simulink model "PV_RT_PI_2017b"  (R2017b)
settings: Solver=ode23tb  StartTime=0.0  StopTime=30  FixedStep=0.01  RelTol=1e-3
values from neighbouring files (symbols this model uses):
  a1 = 900    [LFC_PV_Test_System_Parameters.m]
  B1 = 0.8    [LFC_PV_Test_System_Parameters.m]
  b1 = -18    [LFC_PV_Test_System_Parameters.m]
  c1 = 100    [LFC_PV_Test_System_Parameters.m]
  d1 = 50    [LFC_PV_Test_System_Parameters.m]
  Kps1 = 120    [LFC_PV_Test_System_Parameters.m]
  Kr1 = 0.33    [LFC_PV_Test_System_Parameters.m]
  R1 = 2.5    [LFC_PV_Test_System_Parameters.m]
  T12 = 0.545    [LFC_PV_Test_System_Parameters.m]
  Tg1 = 0.08    [LFC_PV_Test_System_Parameters.m]
  Tps1 = 20    [LFC_PV_Test_System_Parameters.m]
  Tr1 = 10    [LFC_PV_Test_System_Parameters.m]
  Tt1 = 0.3    [LFC_PV_Test_System_Parameters.m]
undefined symbols (not defined in the file or in its folder): Kd, Ki1, Ki2, Kp1, Kp2
libraries: simulink x2
settings Model: Creator=Fujitsu  LastModifiedBy=bora_
settings SolverCC: ZeroCrossAlgorithm=Adaptive
settings DataIOCC: MaxDataPoints=10  SaveFormat=Array  SaveOutput=off  SignalLogging=off  DSMLogging=off  SaveTime=off
settings OptimizationCC: EfficientMapNaN2IntZero=off
settings HardwareCC: TargetBitPerPointer=64  TargetBitPerSizeT=64  TargetBitPerPtrDiffT=64  TargetLongLongMode=on  TargetIntDivRoundTo=Zero  TargetEndianess=LittleEndian  TargetWordSize=64  TargetHWDeviceType=MATLAB Host  ProdEqTarget=off
settings CodeAppCC: MaxIdLength=128
settings GRTTargetCC: TargetLangStandard=C89/C90 (ANSI)  CombineOutputUpdateFcns=off  GRTInterface=on

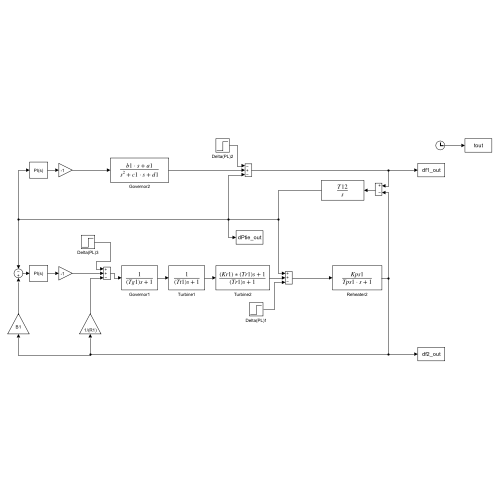
[thumbnail: Simulink's stored preview of the top-level diagram]
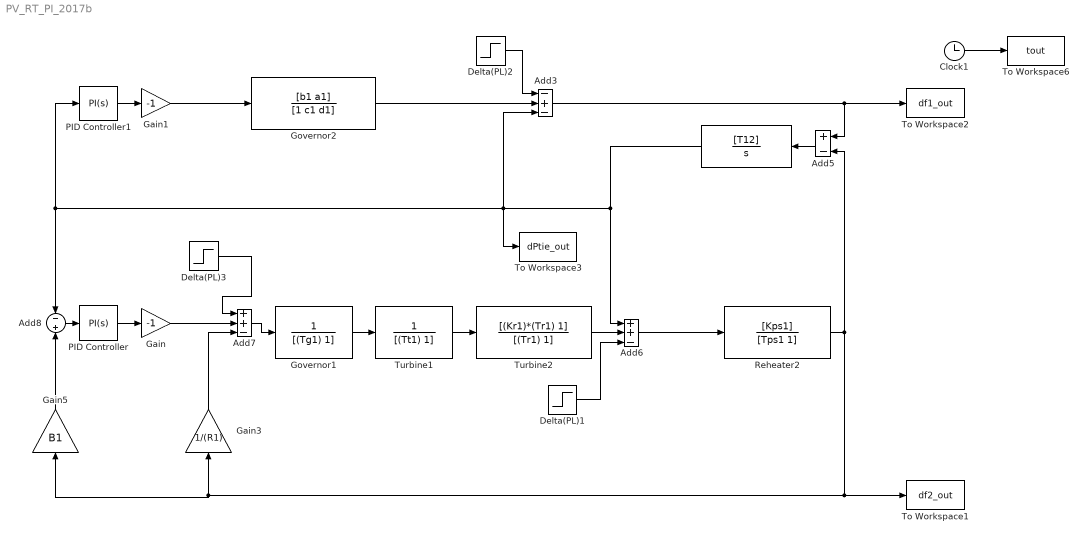
== system PV_RT_PI_2017b ==
  " " : TransferFcn  Numerator=[T12]  Denominator=[1 0]
  Add3 : Sum  Inputs=-+-
  Add5 : Sum  Inputs=+-
  Add6 : Sum  Inputs=++-
  Add7 : Sum  Inputs=++-
  Add8 : Sum  Inputs=-+
  Clock1 : Clock
  Delta(PL)1 : Step  Time=0  After=0.1  SampleTime=0.01
  Delta(PL)2 : Step  Time=0  After=0  SampleTime=0.01
  Delta(PL)3 : Step  Time=0  After=0  SampleTime=0.01
  Gain : Gain  Gain=-1
  Gain1 : Gain  Gain=-1
  Gain3 : Gain  Gain=1/(R1)
  Gain5 : Gain  Gain=B1
  Governor1 : TransferFcn  Denominator=[(Tg1) 1]
  Governor2 : TransferFcn  Numerator=[b1 a1]  Denominator=[1 c1 d1]
  PID Controller : simulink/Continuous/PID Controller  Controller=PI  Form=Parallel  TimeDomain=Continuous-time  SampleTime=-1  IntegratorMethod=Forward Euler  ControllerParametersSource=internal  P=Kp2  I=Ki2  D=Kd  N=10000000  UseFilter=on  TunerSelectOption=Transfer Function Based (PID Tuner App)  InitialConditionSource=internal  InitialConditionForIntegrator=0  InitialConditionForFilter=0  DifferentiatorICPrevScaledInput=0  ExternalReset=none  TrackingMode=off  Kt=1  LimitOutput=off  UpperSaturationLimit=inf  LowerSaturationLimit=-inf  LinearizeAsGain=on  AntiWindupMode=none  Kb=1  POutMin=[]  POutMax=[]  IOutMin=[]  IOutMax=[]  DOutMin=[]  DOutMax=[]  NOutMin=[]  NOutMax=[]  SumOutMin=[]  SumOutMax=[]  SaturationOutMin=[]  SaturationOutMax=[]  PParamMin=[]  PParamMax=[]  IParamMin=[]  IParamMax=[]  DParamMin=[]  DParamMax=[]  NParamMin=[]  NParamMax=[]  KbParamMin=[]  KbParamMax=[]  KtParamMin=[]  KtParamMax=[]  KbOutMin=[]  KbOutMax=[]  KtOutMin=[]  KtOutMax=[]  IntegratorOutMin=[]  IntegratorOutMax=[]  FilterOutMin=[]  FilterOutMax=[]  SumI1OutMin=[]  SumI1OutMax=[]  SumI2OutMin=[]  SumI2OutMax=[]  SumI3OutMin=[]  SumI3OutMax=[]  SumDOutMin=[]  SumDOutMax=[]  DifferentiatorOutMin=[]  DifferentiatorOutMax=[]  FilterDiffOutCoefMin=[]  FilterDiffOutCoefMax=[]  ReciprocalOutMin=[]  ReciprocalOutMax=[]  SumDenOutMin=[]  SumDenOutMax=[]  SumNumOutMin=[]  SumNumOutMax=[]  DivideOutMin=[]  DivideOutMax=[]  IntegratorContinuousStateAttributes=''  IntegratorStateMustResolveToSignalObject=off  IntegratorRTWStateStorageClass=Auto  FilterContinuousStateAttributes=''  FilterStateMustResolveToSignalObject=off  FilterRTWStateStorageClass=Auto  InitialConditionSetting=State (most efficient)
  PID Controller1 : simulink/Continuous/PID Controller  Controller=PI  Form=Parallel  TimeDomain=Continuous-time  SampleTime=-1  IntegratorMethod=Forward Euler  ControllerParametersSource=internal  P=Kp1  I=Ki1  D=Kd  N=1000000  UseFilter=on  TunerSelectOption=Transfer Function Based (PID Tuner App)  InitialConditionSource=internal  InitialConditionForIntegrator=0  InitialConditionForFilter=0  DifferentiatorICPrevScaledInput=0  ExternalReset=none  TrackingMode=off  Kt=1  LimitOutput=off  UpperSaturationLimit=inf  LowerSaturationLimit=-inf  LinearizeAsGain=on  AntiWindupMode=none  Kb=1  POutMin=[]  POutMax=[]  IOutMin=[]  IOutMax=[]  DOutMin=[]  DOutMax=[]  NOutMin=[]  NOutMax=[]  SumOutMin=[]  SumOutMax=[]  SaturationOutMin=[]  SaturationOutMax=[]  PParamMin=[]  PParamMax=[]  IParamMin=[]  IParamMax=[]  DParamMin=[]  DParamMax=[]  NParamMin=[]  NParamMax=[]  KbParamMin=[]  KbParamMax=[]  KtParamMin=[]  KtParamMax=[]  KbOutMin=[]  KbOutMax=[]  KtOutMin=[]  KtOutMax=[]  IntegratorOutMin=[]  IntegratorOutMax=[]  FilterOutMin=[]  FilterOutMax=[]  SumI1OutMin=[]  SumI1OutMax=[]  SumI2OutMin=[]  SumI2OutMax=[]  SumI3OutMin=[]  SumI3OutMax=[]  SumDOutMin=[]  SumDOutMax=[]  DifferentiatorOutMin=[]  DifferentiatorOutMax=[]  FilterDiffOutCoefMin=[]  FilterDiffOutCoefMax=[]  ReciprocalOutMin=[]  ReciprocalOutMax=[]  SumDenOutMin=[]  SumDenOutMax=[]  SumNumOutMin=[]  SumNumOutMax=[]  DivideOutMin=[]  DivideOutMax=[]  IntegratorContinuousStateAttributes=''  IntegratorStateMustResolveToSignalObject=off  IntegratorRTWStateStorageClass=Auto  FilterContinuousStateAttributes=''  FilterStateMustResolveToSignalObject=off  FilterRTWStateStorageClass=Auto  InitialConditionSetting=State (most efficient)
  Reheater2 : TransferFcn  Numerator=[Kps1]  Denominator=[Tps1 1]
  To Workspace1 : ToWorkspace  VariableName=df2_out  SampleTime=0.01
  To Workspace2 : ToWorkspace  VariableName=df1_out  SampleTime=0.01
  To Workspace3 : ToWorkspace  VariableName=dPtie_out  SampleTime=0.01
  To Workspace6 : ToWorkspace  VariableName=tout  SampleTime=0.01
  Turbine1 : TransferFcn  Denominator=[(Tt1) 1]
  Turbine2 : TransferFcn  Numerator=[(Kr1)*(Tr1) 1]  Denominator=[(Tr1) 1]
  wires:
  " "/1 -> Add6/1, To Workspace3/1, Add3/3, PID Controller1/1, Add8/1
  Gain5/1 -> Add8/2
  Reheater2/1 -> Gain5/1, Gain3/1, To Workspace1/1, Add5/2
  Gain3/1 -> Add7/3
  Delta(PL)1/1 -> Add6/3
  Turbine1/1 -> Turbine2/1
  Governor1/1 -> Turbine1/1
  Add5/1 -> " "/1
  Add7/1 -> Governor1/1
  Turbine2/1 -> Add6/2
  PID Controller1/1 -> Gain1/1
  Governor2/1 -> Add3/2
  Delta(PL)2/1 -> Add3/1
  Add8/1 -> PID Controller/1
  PID Controller/1 -> Gain/1
  Delta(PL)3/1 -> Add7/1
  Gain1/1 -> Governor2/1
  Gain/1 -> Add7/2
  Add3/1 -> Add5/1, To Workspace2/1
  Add6/1 -> Reheater2/1
  Clock1/1 -> To Workspace6/1
